simulink model "task3"  (R2023b)
settings: Solver=FixedStepDiscrete  StartTime=0.0  StopTime=60*10  FixedStep=5e-5  RelTol=1e-3
PreLoadFcn:
  | Simulink.defineIntEnumType('windowCommand', {'Off','Speed1','Speed2','Speed3'},[0,1,2,3])
libraries: simulink x4
settings Model: Creator=kz1nz0  LastModifiedBy=kaynt

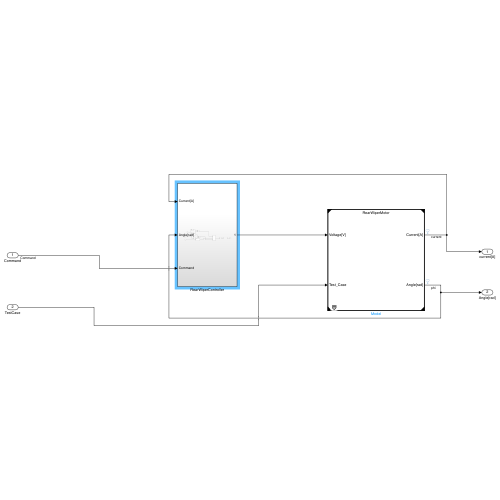
[thumbnail: Simulink's stored preview of the top-level diagram]
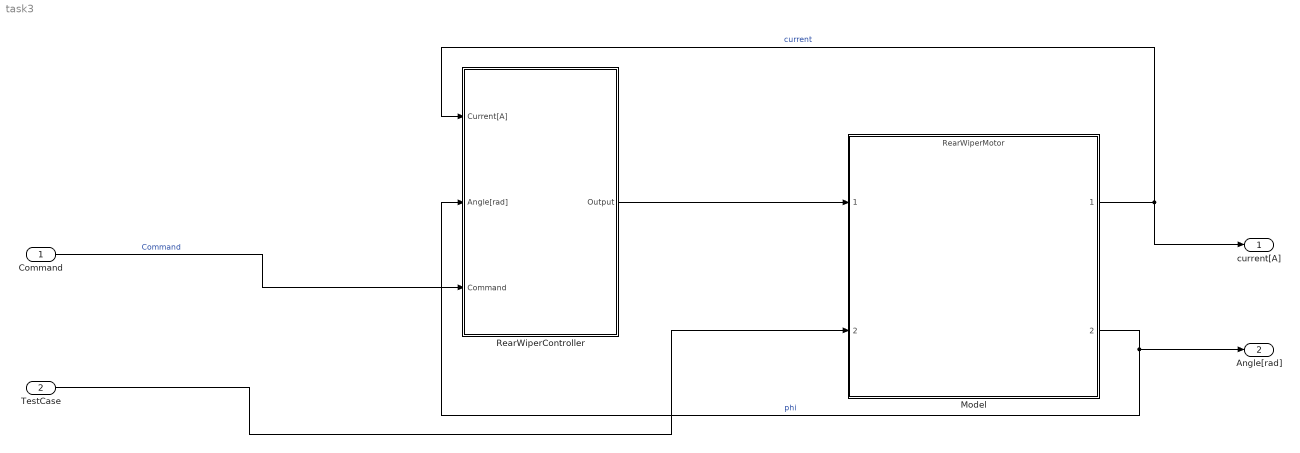
== system task3 ==
  Command : Inport  OutDataTypeStr=Enum: windowCommand
  TestCase : Inport  Port=2  OutDataTypeStr=int8
  Model : ModelReference  ModelNameDialog=RearWiperMotor.slxp  ModelReferenceVersion=19.15  CopyOfModelProtected=on
  RearWiperController : Subsystem
  current[A] : Outport
  Angle[rad] : Outport  Port=2
  wires:
  Command/1 -> RearWiperController/3(Command)  "Command"
  TestCase/1 -> Model/2
  Model/1 -> current[A]/1, RearWiperController/1(Current[A])  "current"
  Model/2 -> RearWiperController/2(Angle[rad]), Angle[rad]/1  "phi"
  RearWiperController/1(Output) -> Model/1

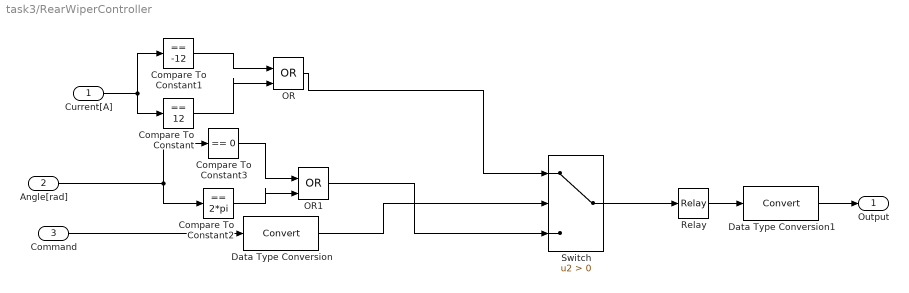
== system task3/RearWiperController ==
  Current[A] : Inport
  Angle[rad] : Inport  Port=2
  Command : Inport  Port=3  OutDataTypeStr=Enum: windowCommand
  Compare To Constant : simulink/Logic and Bit Operations/Compare To Constant  relop===  const=12  OutDataTypeStr=boolean
  Compare To Constant1 : simulink/Logic and Bit Operations/Compare To Constant  relop===  const=-12  OutDataTypeStr=boolean
  Compare To Constant2 : simulink/Logic and Bit Operations/Compare To Constant  relop===  const=2*pi  OutDataTypeStr=boolean
  Compare To Constant3 : simulink/Logic and Bit Operations/Compare To Constant  relop===  const=0  OutDataTypeStr=boolean
  Data Type Conversion : DataTypeConversion  SaturateOnIntegerOverflow=off  RndMeth=Floor
  Data Type Conversion1 : DataTypeConversion  SaturateOnIntegerOverflow=off  RndMeth=Floor
  OR : Logic  Operator=OR  IconShape=distinctive  AllPortsSameDT=off  OutDataTypeStr=boolean
  OR1 : Logic  Operator=OR  IconShape=distinctive  AllPortsSameDT=off  OutDataTypeStr=boolean
  Relay : Relay  OnSwitchValue=1  OffSwitchValue=0  OnOutputValue=12  OffOutputValue=-12
  Switch : Switch  Criteria=u2 > Threshold  SaturateOnIntegerOverflow=off  InputSameDT=off
  Output : Outport
  wires:
  Current[A]/1 -> Compare To Constant/1, Compare To Constant1/1
  Compare To Constant/1 -> OR/2
  Compare To Constant1/1 -> OR/1
  Compare To Constant3/1 -> OR1/1
  Compare To Constant2/1 -> OR1/2
  Command/1 -> Data Type Conversion/1
  Angle[rad]/1 -> Compare To Constant3/1, Compare To Constant2/1
  OR/1 -> Switch/1
  OR1/1 -> Switch/3
  Switch/1 -> Relay/1
  Data Type Conversion/1 -> Switch/2
  Relay/1 -> Data Type Conversion1/1
  Data Type Conversion1/1 -> Output/1
